simulink model "hexapod2"  (R2015a)
settings: Solver=ode23tb  StartTime=0.0  StopTime=10  FixedStep=0.0001  MaxStep=0.01  RelTol=1e-4  AbsTol=1e-5
values from neighbouring files (symbols this model uses):
  bH = 1    [runFirst.m]
  C = CM + CL/n^2    (= 0.0001377500155)    [runFirst.m]
  d1 = 0    [runFirst.m]    (also in runFirst2.m)
  d2 = -4.61    [runFirst.m]    (also in runFirst2.m = 0)
  J = JM + JL/n^2    (= 0.008455500031)    [runFirst.m]
  Ka = 12    [runFirst.m]
  Kb = 0.00867    [runFirst.m]
  Ke = 1    [runFirst.m]
  Km = 4.375    [runFirst.m]
  L = 0.0006    [runFirst.m]
  L1 = 3.64    [runFirst.m]    (also in runFirst2.m = 3.4)
  L2 = 5.72    [runFirst.m]    (also in runFirst2.m = 8.7)
  L3 = 12.46    [runFirst.m]    (also in runFirst2.m = 12.73)
  n = 254    [runFirst.m]
  R = 1.4    [runFirst.m]
undefined symbols (not defined in the file or in its folder): bLb, bLs, X, Y, Z
libraries: sm_lib x108, nesl_utility x43, simulink x24, Contact_Forces_Lib x7, roblocks x2
(part 1 of 5)
settings Model: Creator=340DANILOV  LastModifiedBy=340DANILOV
settings SolverCC: ZeroCrossAlgorithm=Adaptive
settings DataIOCC: LimitDataPoints=off  ReturnWorkspaceOutputs=on
settings DebuggingCC: IgnoredZcDiagnostic=none  SolverPrmCheckMsg=warning  UnconnectedInputMsg=none  UnconnectedOutputMsg=none
settings DiagnosticsConfigSet: SimMechanicsRigidlyBoundBlock=none

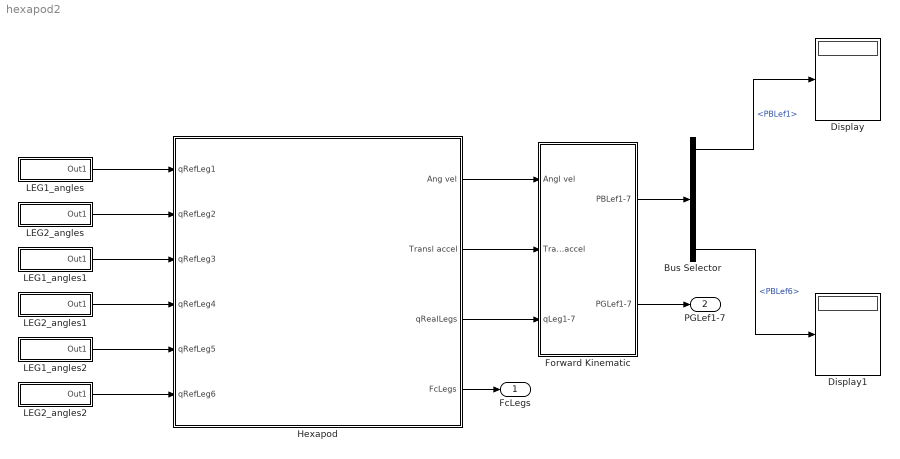
== system hexapod2 ==
  Bus Selector : BusSelector  OutputSignals=PBLef1,PBLef2,PBLef3,PBLef4,PBLef5,PBLef6
  Display : Display
  Display1 : Display
  Forward Kinematic : Subsystem
  Hexapod : Subsystem  mask(Hexapod model){}
      mask help:
      | This model describes hexapod robot with six insect legs. This model contain mechanics and servos.
      | You can change mass and size charasteristics of body and legs.
      | As a location is used a flat surface.
      |
      | Inputs:
      |  - qRefLeg<1...6> - reference angles for each leg.
      |             It is must be 1x3 massive with angles for each joint of leg.
      |
      | Outputs:
      |  - Ang vel - Angular velocities of CoM. Imitation of data from gyroscope.
      |  - Transl accel - CoM translation acceleration. Imitation of data from accelerometer.
      |  - FcLegs - Contact forces of end effectors each leg. It is 1x6 massive. Each element contains value for contact force each leg. Imitation of force sensors.
      |  - qRealLegs - Real angles of each link of hexapod legs. It is 3x6 massive. Imitation of data from servo encoder.
      mask Display:
      | image(imread('hexapod.png'))
      | 
      | 
      | port_label('output',1,'Ang vel')
      | port_label('output',2,'Transl accel')
      | port_label('output',3,'qRealLegs')
      | port_label('output',4,'FcLegs')
      | 
      | port_label('input',1,'qRefLeg1')
      | port_label('input',2,'qRefLeg2')
      | port_label('input',3,'qRefLeg3')
      | port_label('input',4,'qRefLeg4')
      | port_label('input',5,'qRefLeg5')
      | port_label('input',6,'qRefLeg6')
  LEG1_angles : Subsystem
  LEG1_angles1 : Subsystem
  LEG1_angles2 : Subsystem
  LEG2_angles : Subsystem
  LEG2_angles1 : Subsystem
  LEG2_angles2 : Subsystem
  FcLegs : Outport
  PGLef1-7 : Outport  Port=2
  wires:
  Hexapod/4(FcLegs) -> FcLegs/1
  Hexapod/1(Ang vel) -> Forward Kinematic/1(Angl vel)
  Hexapod/2(Transl accel) -> Forward Kinematic/2(Transl accel)
  Hexapod/3(qRealLegs) -> Forward Kinematic/3(qLeg1-7)
  Forward Kinematic/1(PBLef1-7) -> Bus Selector/1
  Forward Kinematic/2(PGLef1-7) -> PGLef1-7/1
  Bus Selector/1 -> Display/1  "<PBLef1>"
  Bus Selector/6 -> Display1/1  "<PBLef6>"
  LEG1_angles/1(Out1) -> Hexapod/1(qRefLeg1)
  LEG2_angles/1(Out1) -> Hexapod/2(qRefLeg2)
  LEG2_angles1/1(Out1) -> Hexapod/4(qRefLeg4)
  LEG2_angles2/1(Out1) -> Hexapod/6(qRefLeg6)
  LEG1_angles1/1(Out1) -> Hexapod/3(qRefLeg3)
  LEG1_angles2/1(Out1) -> Hexapod/5(qRefLeg5)

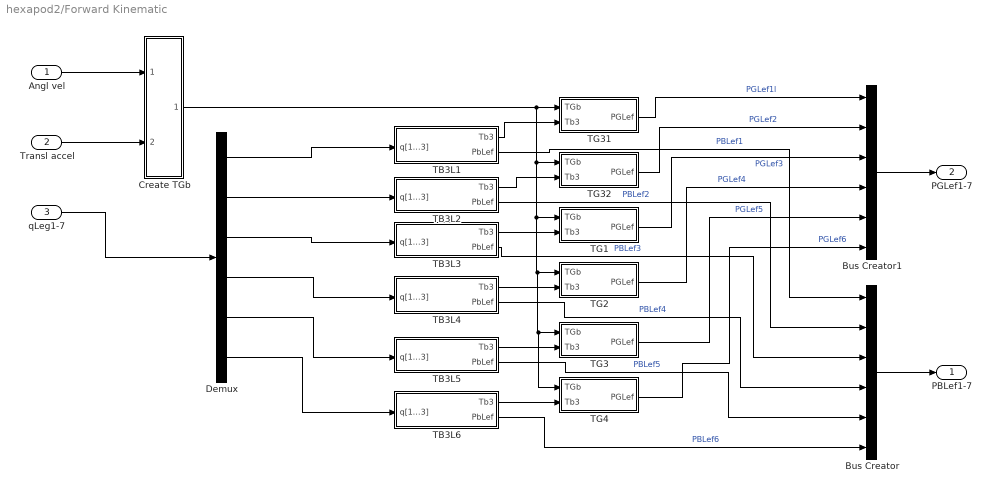
== system hexapod2/Forward Kinematic ==
  Angl vel : Inport
  Transl accel : Inport  Port=2
  qLeg1-7 : Inport  Port=3
  Bus Creator : BusCreator  Inputs=6
  Bus Creator1 : BusCreator  Inputs=6
  Create TGb : Subsystem
  Demux : Demux  Outputs=6
  TB3L1 : Subsystem
  TB3L2 : Subsystem
  TB3L3 : Subsystem
  TB3L4 : Subsystem
  TB3L5 : Subsystem
  TB3L6 : Subsystem
  TG1 : Subsystem
  TG2 : Subsystem
  TG3 : Subsystem
  TG31 : Subsystem
  TG32 : Subsystem
  TG4 : Subsystem
  PBLef1-7 : Outport
  PGLef1-7 : Outport  Port=2
  wires:
  Bus Creator/1 -> PBLef1-7/1
  TB3L6/1(Tb3) -> TG4/2(Tb3)
  TB3L5/2(PbLef) -> Bus Creator/5  "PBLef5"
  TB3L4/2(PbLef) -> Bus Creator/4  "PBLef4"
  TG3/1(PGLef) -> Bus Creator1/5  "PGLef5"
  TB3L6/2(PbLef) -> Bus Creator/6  "PBLef6"
  Demux/1 -> TB3L1/1(q[1...3])
  TB3L1/2(PbLef) -> Bus Creator/1  "PBLef1"
  Demux/6 -> TB3L6/1(q[1...3])
  TB3L1/1(Tb3) -> TG31/2(Tb3)
  Create TGb/1(Out1) -> TG4/1(TGb), TG3/1(TGb), TG2/1(TGb), TG1/1(TGb), TG32/1(TGb), TG31/1(TGb)
  Demux/4 -> TB3L4/1(q[1...3])
  Demux/3 -> TB3L3/1(q[1...3])
  TG31/1(PGLef) -> Bus Creator1/1  "PGLef1l"
  Demux/5 -> TB3L5/1(q[1...3])
  TB3L2/2(PbLef) -> Bus Creator/2  "PBLef2"
  TB3L2/1(Tb3) -> TG32/2(Tb3)
  TG32/1(PGLef) -> Bus Creator1/2  "PGLef2"
  TB3L4/1(Tb3) -> TG2/2(Tb3)
  TB3L3/1(Tb3) -> TG1/2(Tb3)
  TG1/1(PGLef) -> Bus Creator1/3  "PGLef3"
  Bus Creator1/1 -> PGLef1-7/1
  Angl vel/1 -> Create TGb/1(In1)
  Transl accel/1 -> Create TGb/2(In2)
  TB3L3/2(PbLef) -> Bus Creator/3  "PBLef3"
  qLeg1-7/1 -> Demux/1
  TB3L5/1(Tb3) -> TG3/2(Tb3)
  TG4/1(PGLef) -> Bus Creator1/6  "PGLef6"
  TG2/1(PGLef) -> Bus Creator1/4  "PGLef4"
  Demux/2 -> TB3L2/1(q[1...3])

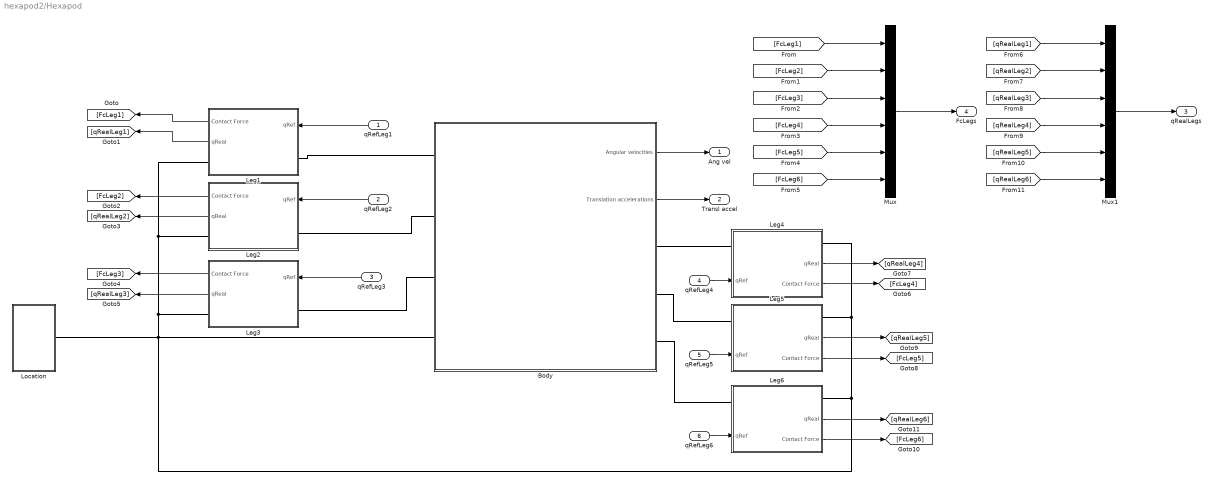
== system hexapod2/Hexapod ==
  qRefLeg1 : Inport
  qRefLeg2 : Inport  Port=2
  qRefLeg3 : Inport  Port=3
  qRefLeg4 : Inport  Port=4
  qRefLeg5 : Inport  Port=5
  qRefLeg6 : Inport  Port=6
  Body : Subsystem  mask(Hexapod Body){L=18.5, w1=10.5, w2=12.5, H=1, m=5, Z1Angle=45, Z2Angle=0, Z3Angle=-45, Z4Angle=-45, Z5Angle=0, Z6Angle=45}
      mask prompts: L "Length (cm)"; w1 "Small weigth (cm)"; w2 "Big weigth (cm)"; H "Heigth (cm)"; m "Mass (kg)"; Z1Angle "Leg1 Rotation"; Z2Angle "Leg2 Rotation"; Z3Angle "Leg3 Rotation"; Z4Angle "Leg4 Rotation"; Z5Angle "Leg5 Rotation"; Z6Angle "Leg6 Rotation"
      mask help: This block describes overall size, mass and reference frames of hexapod body.
      mask Display:
      | image(imread('body.png'))
      | text(5,10, 'Hexapod Body')
      | port_label('LConn',1,'Leg1')
      | port_label('LConn',2,'Leg2')
      | port_label('LConn',3,'Leg3')
      | port_label('LConn',4,'Global System')
      | port_label('RConn',1,'Leg4')
      | port_label('RConn',2,'Leg5')
      | port_label('RConn',3,'Leg6')
      | port_label('output',1,'Ang vel')
      | port_label('output',2,'Transl accel')
  Leg1 : Subsystem  mask(Insect leg){L1=L1, L2=L2, L3=L3, m1=0.1, m2=0.1, m3=0.1}
      mask prompts: L1 "Length 1 (cm)"; L2 "Lengh 2 (cm)"; L3 "Length 3 (cm)"; m1 "Mass 1 (kg)"; m2 "Mass 2 (kg)"; m3 "Mass 3(kg)"
      mask help: This block describes link length and their mass of the hexapod insect leg.
      mask Display:
      | image(imread('insect_leg.png'))
      | text(5,10, 'Insect leg')
      | port_label('LConn',1,'T0')
      | port_label('RConn',1,'Base')
      | port_label('input',1,'qRef')
      | port_label('output',1,'Fc')
      | port_label('output',2,'qReal')
  Leg2 : Subsystem  mask(Insect leg){L1=3.53, L2=5.7, L3=12.6, m1=0.1, m2=0.1, m3=0.1}
      mask prompts: L1 "Length 1 (cm)"; L2 "Lengh 2 (cm)"; L3 "Length 3 (cm)"; m1 "Mass 1 (kg)"; m2 "Mass 2 (kg)"; m3 "Mass 3(kg)"
      mask help: This block describes link length and their mass of the hexapod insect leg.
      mask Display:
      | image(imread('insect_leg.png'))
      | text(5,10, 'Insect leg')
      | port_label('LConn',1,'T0')
      | port_label('RConn',1,'Base')
      | port_label('input',1,'qRef')
      | port_label('output',1,'Fc')
      | port_label('output',2,'qReal')
  Leg3 : Subsystem  mask(Insect leg){L1=3.53, L2=5.7, L3=12.6, m1=0.1, m2=0.1, m3=0.1}
      mask prompts: L1 "Length 1 (cm)"; L2 "Lengh 2 (cm)"; L3 "Length 3 (cm)"; m1 "Mass 1 (kg)"; m2 "Mass 2 (kg)"; m3 "Mass 3(kg)"
      mask help: This block describes link length and their mass of the hexapod insect leg.
      mask Display:
      | image(imread('insect_leg.png'))
      | text(5,10, 'Insect leg')
      | port_label('LConn',1,'T0')
      | port_label('RConn',1,'Base')
      | port_label('input',1,'qRef')
      | port_label('output',1,'Fc')
      | port_label('output',2,'qReal')
  Leg4 : Subsystem  mask(Insect leg){L1=3.53, L2=5.7, L3=12.6, m1=0.1, m2=0.1, m3=0.1}
      mask prompts: L1 "Length 1 (cm)"; L2 "Lengh 2 (cm)"; L3 "Length 3 (cm)"; m1 "Mass 1 (kg)"; m2 "Mass 2 (kg)"; m3 "Mass 3(kg)"
      mask help: This block describes link length and their mass of the hexapod insect leg.
      mask Display:
      | image(imread('insect_leg.png'))
      | text(5,10, 'Insect leg')
      | port_label('LConn',1,'T0')
      | port_label('RConn',1,'Base')
      | port_label('input',1,'qRef')
      | port_label('output',1,'Fc')
      | port_label('output',2,'qReal')
  Leg5 : Subsystem  mask(Insect leg){L1=3.53, L2=5.7, L3=12.6, m1=0.1, m2=0.1, m3=0.1}
      mask prompts: L1 "Length 1 (cm)"; L2 "Lengh 2 (cm)"; L3 "Length 3 (cm)"; m1 "Mass 1 (kg)"; m2 "Mass 2 (kg)"; m3 "Mass 3(kg)"
      mask help: This block describes link length and their mass of the hexapod insect leg.
      mask Display:
      | image(imread('insect_leg.png'))
      | text(5,10, 'Insect leg')
      | port_label('LConn',1,'T0')
      | port_label('RConn',1,'Base')
      | port_label('input',1,'qRef')
      | port_label('output',1,'Fc')
      | port_label('output',2,'qReal')
  Leg6 : Subsystem  mask(Insect leg){L1=3.53, L2=5.7, L3=12.6, m1=0.1, m2=0.1, m3=0.1}
      mask prompts: L1 "Length 1 (cm)"; L2 "Lengh 2 (cm)"; L3 "Length 3 (cm)"; m1 "Mass 1 (kg)"; m2 "Mass 2 (kg)"; m3 "Mass 3(kg)"
      mask help: This block describes link length and their mass of the hexapod insect leg.
      mask Display:
      | image(imread('insect_leg.png'))
      | text(5,10, 'Insect leg')
      | port_label('LConn',1,'T0')
      | port_label('RConn',1,'Base')
      | port_label('input',1,'qRef')
      | port_label('output',1,'Fc')
      | port_label('output',2,'qReal')
  Location : Subsystem
  Mux : Mux  Inputs=6
  Mux1 : Mux  Inputs=6
  Ang vel : Outport
  Transl accel : Outport  Port=2
  qRealLegs : Outport  Port=3
  FcLegs : Outport  Port=4
  wires:
  qRefLeg1/1 -> Leg1/1(qRef)
  qRefLeg2/1 -> Leg2/1(qRef)
  qRefLeg3/1 -> Leg3/1(qRef)
  qRefLeg4/1 -> Leg4/1(qRef)
  Leg2/2(qReal) -> [qRealLeg2]
  Leg3/2(qReal) -> [qRealLeg3]
  Leg3/1(Contact Force) -> [FcLeg3]
  [FcLeg2] -> Mux/2
  [FcLeg4] -> Mux/4
  [FcLeg5] -> Mux/5
  [FcLeg1] -> Mux/1
  [FcLeg3] -> Mux/3
  [FcLeg6] -> Mux/6
  Mux/1 -> FcLegs/1
  Leg1/1(Contact Force) -> [FcLeg1]
  [qRealLeg4] -> Mux1/4
  [qRealLeg6] -> Mux1/6
  [qRealLeg2] -> Mux1/2
  [qRealLeg1] -> Mux1/1
  Mux1/1 -> qRealLegs/1
  [qRealLeg5] -> Mux1/5
  [qRealLeg3] -> Mux1/3
  Body/1(Angular velocities) -> Ang vel/1
  Body/2(Translation accelerations) -> Transl accel/1
  Leg1/2(qReal) -> [qRealLeg1]
  Leg2/1(Contact Force) -> [FcLeg2]
  qRefLeg5/1 -> Leg5/1(qRef)
  qRefLeg6/1 -> Leg6/1(qRef)
  Leg4/1(Contact Force) -> [FcLeg4]
  Leg4/2(qReal) -> [qRealLeg4]
  Leg5/2(qReal) -> [qRealLeg5]
  Leg5/1(Contact Force) -> [FcLeg5]
  Leg6/2(qReal) -> [qRealLeg6]
  Leg6/1(Contact Force) -> [FcLeg6]
  connections:
  Body/LConn1 -- Leg1/LConn1
  Body/LConn4 -- Leg6/RConn1 -- Leg5/RConn1 -- Leg4/RConn1 -- Location/RConn1 -- Leg3/RConn1 -- Leg2/RConn1 -- Leg1/RConn1
  Leg2/LConn1 -- Body/LConn2
  Leg3/LConn1 -- Body/LConn3
  Leg4/LConn1 -- Body/RConn1
  Leg5/LConn1 -- Body/RConn2
  Leg6/LConn1 -- Body/RConn3

== system hexapod2/LEG1_angles ==
  Clock : Clock
  Mux : Mux  Inputs=3
  Switch : Switch  Threshold=6
  leg1_theta2 : simulink/Sources/Repeating Sequence  rep_seq_t=[0 3 4 5 6]  rep_seq_y=[0 0 60*pi/180 60*pi/180 0]
  leg1_theta3 : simulink/Sources/Repeating Sequence  rep_seq_t=[0 3 4 5 6]  rep_seq_y=[0 0 60*pi/180 60*pi/180 0]
  theta1 : simulink/Sources/Repeating Sequence Interpolated  OutValues=[0 0 0 45*pi/180 45*pi/180].'  TimeValues=[0 3 4 5 6].'  LookUpMeth=Interpolation-Use End Values  tsamp=0.01  OutMin=[]  OutMax=[]  OutDataTypeStr=double  OutputDataTypeScalingMode=double  OutDataType=fixdt(0,8)  OutScaling=2^-10
  theta21 : simulink/Sources/Repeating Sequence Interpolated  OutValues=[45*pi/180 -45*pi/180 -45*pi/180 45*pi/180 45*pi/180].'  TimeValues=[0 3 4 5 6].'  LookUpMeth=Interpolation-Use End Values  tsamp=0.01  OutMin=[]  OutMax=[]  OutDataTypeStr=double  OutputDataTypeScalingMode=double  OutDataType=fixdt(0,8)  OutScaling=2^-10
  Out1 : Outport
  wires:
  theta1/1 -> Switch/3
  theta21/1 -> Switch/1
  Switch/1 -> Mux/1
  Clock/1 -> Switch/2
  Mux/1 -> Out1/1
  leg1_theta3/1 -> Mux/3
  leg1_theta2/1 -> Mux/2

== system hexapod2/LEG1_angles1 ==
  Clock : Clock
  Mux : Mux  Inputs=3
  Switch : Switch  Threshold=6
  leg1_theta2 : simulink/Sources/Repeating Sequence  rep_seq_t=[0 3 4 5 6]  rep_seq_y=[0 0 60*pi/180 60*pi/180 0]
  leg1_theta3 : simulink/Sources/Repeating Sequence  rep_seq_t=[0 3 4 5 6]  rep_seq_y=[0 0 60*pi/180 60*pi/180 0]
  theta1 : simulink/Sources/Repeating Sequence Interpolated  OutValues=[0 0 0 45*pi/180 45*pi/180].'  TimeValues=[0 3 4 5 6].'  LookUpMeth=Interpolation-Use End Values  tsamp=0.01  OutMin=[]  OutMax=[]  OutDataTypeStr=double  OutputDataTypeScalingMode=double  OutDataType=fixdt(0,8)  OutScaling=2^-10
  theta21 : simulink/Sources/Repeating Sequence Interpolated  OutValues=[45*pi/180 -45*pi/180 -45*pi/180 45*pi/180 45*pi/180].'  TimeValues=[0 3 4 5 6].'  LookUpMeth=Interpolation-Use End Values  tsamp=0.01  OutMin=[]  OutMax=[]  OutDataTypeStr=double  OutputDataTypeScalingMode=double  OutDataType=fixdt(0,8)  OutScaling=2^-10
  Out1 : Outport
  wires:
  leg1_theta2/1 -> Mux/2
  leg1_theta3/1 -> Mux/3
  Mux/1 -> Out1/1
  Clock/1 -> Switch/2
  Switch/1 -> Mux/1
  theta21/1 -> Switch/1
  theta1/1 -> Switch/3

== system hexapod2/LEG1_angles2 ==
  Clock : Clock
  Mux : Mux  Inputs=3
  Switch : Switch  Threshold=6
  leg1_theta2 : simulink/Sources/Repeating Sequence  rep_seq_t=[0 3 4 5 6]  rep_seq_y=[0 0 60*pi/180 60*pi/180 0]
  leg1_theta3 : simulink/Sources/Repeating Sequence  rep_seq_t=[0 3 4 5 6]  rep_seq_y=[0 0 60*pi/180 60*pi/180 0]
  theta1 : simulink/Sources/Repeating Sequence Interpolated  OutValues=[0 0 0 45*pi/180 45*pi/180].'  TimeValues=[0 3 4 5 6].'  LookUpMeth=Interpolation-Use End Values  tsamp=0.01  OutMin=[]  OutMax=[]  OutDataTypeStr=double  OutputDataTypeScalingMode=double  OutDataType=fixdt(0,8)  OutScaling=2^-10
  theta21 : simulink/Sources/Repeating Sequence Interpolated  OutValues=[45*pi/180 -45*pi/180 -45*pi/180 45*pi/180 45*pi/180].'  TimeValues=[0 3 4 5 6].'  LookUpMeth=Interpolation-Use End Values  tsamp=0.01  OutMin=[]  OutMax=[]  OutDataTypeStr=double  OutputDataTypeScalingMode=double  OutDataType=fixdt(0,8)  OutScaling=2^-10
  Out1 : Outport
  wires:
  theta1/1 -> Switch/3
  theta21/1 -> Switch/1
  Switch/1 -> Mux/1
  Clock/1 -> Switch/2
  Mux/1 -> Out1/1
  leg1_theta3/1 -> Mux/3
  leg1_theta2/1 -> Mux/2

== system hexapod2/LEG2_angles ==
  Clock : Clock
  Mux1 : Mux  Inputs=3
  Switch : Switch  Threshold=6
  leg2_theta2 : simulink/Sources/Repeating Sequence  rep_seq_t=[0 1 2 3 6]  rep_seq_y=[0 60*pi/180 60*pi/180 0 0]
  leg2_theta3 : simulink/Sources/Repeating Sequence  rep_seq_t=[0 1 2 3 6]  rep_seq_y=[0 60*pi/180 60*pi/180 0 0]
  theta1 : simulink/Sources/Repeating Sequence Interpolated  OutValues=[0 0 45*pi/180 45*pi/180 -45*pi/180].'  TimeValues=[0 1 2 3 6].'  LookUpMeth=Interpolation-Use End Values  tsamp=0.01  OutMin=[]  OutMax=[]  OutDataTypeStr=double  OutputDataTypeScalingMode=double  OutDataType=fixdt(0,8)  OutScaling=2^-10
  theta21 : simulink/Sources/Repeating Sequence Interpolated  OutValues=[-45*pi/180 -45*pi/180 45*pi/180 45*pi/180 -45*pi/180].'  TimeValues=[0 1 2 3 6].'  LookUpMeth=Interpolation-Use End Values  tsamp=0.01  OutMin=[]  OutMax=[]  OutDataTypeStr=double  OutputDataTypeScalingMode=double  OutDataType=fixdt(0,8)  OutScaling=2^-10
  Out1 : Outport
  wires:
  Switch/1 -> Mux1/1
  theta1/1 -> Switch/3
  theta21/1 -> Switch/1
  Clock/1 -> Switch/2
  leg2_theta2/1 -> Mux1/2
  leg2_theta3/1 -> Mux1/3
  Mux1/1 -> Out1/1

== system hexapod2/LEG2_angles1 ==
  Clock : Clock
  Mux1 : Mux  Inputs=3
  Switch : Switch  Threshold=6
  leg2_theta2 : simulink/Sources/Repeating Sequence  rep_seq_t=[0 1 2 3 6]  rep_seq_y=[0 60*pi/180 60*pi/180 0 0]
  leg2_theta3 : simulink/Sources/Repeating Sequence  rep_seq_t=[0 1 2 3 6]  rep_seq_y=[0 60*pi/180 60*pi/180 0 0]
  theta1 : simulink/Sources/Repeating Sequence Interpolated  OutValues=[0 0 45*pi/180 45*pi/180 -45*pi/180].'  TimeValues=[0 1 2 3 6].'  LookUpMeth=Interpolation-Use End Values  tsamp=0.01  OutMin=[]  OutMax=[]  OutDataTypeStr=double  OutputDataTypeScalingMode=double  OutDataType=fixdt(0,8)  OutScaling=2^-10
  theta21 : simulink/Sources/Repeating Sequence Interpolated  OutValues=[-45*pi/180 -45*pi/180 45*pi/180 45*pi/180 -45*pi/180].'  TimeValues=[0 1 2 3 6].'  LookUpMeth=Interpolation-Use End Values  tsamp=0.01  OutMin=[]  OutMax=[]  OutDataTypeStr=double  OutputDataTypeScalingMode=double  OutDataType=fixdt(0,8)  OutScaling=2^-10
  Out1 : Outport
  wires:
  Mux1/1 -> Out1/1
  leg2_theta3/1 -> Mux1/3
  leg2_theta2/1 -> Mux1/2
  Clock/1 -> Switch/2
  theta21/1 -> Switch/1
  theta1/1 -> Switch/3
  Switch/1 -> Mux1/1

== system hexapod2/LEG2_angles2 ==
  Clock : Clock
  Mux1 : Mux  Inputs=3
  Switch : Switch  Threshold=6
  leg2_theta2 : simulink/Sources/Repeating Sequence  rep_seq_t=[0 1 2 3 6]  rep_seq_y=[0 60*pi/180 60*pi/180 0 0]
  leg2_theta3 : simulink/Sources/Repeating Sequence  rep_seq_t=[0 1 2 3 6]  rep_seq_y=[0 60*pi/180 60*pi/180 0 0]
  theta1 : simulink/Sources/Repeating Sequence Interpolated  OutValues=[0 0 45*pi/180 45*pi/180 -45*pi/180].'  TimeValues=[0 1 2 3 6].'  LookUpMeth=Interpolation-Use End Values  tsamp=0.01  OutMin=[]  OutMax=[]  OutDataTypeStr=double  OutputDataTypeScalingMode=double  OutDataType=fixdt(0,8)  OutScaling=2^-10
  theta21 : simulink/Sources/Repeating Sequence Interpolated  OutValues=[-45*pi/180 -45*pi/180 45*pi/180 45*pi/180 -45*pi/180].'  TimeValues=[0 1 2 3 6].'  LookUpMeth=Interpolation-Use End Values  tsamp=0.01  OutMin=[]  OutMax=[]  OutDataTypeStr=double  OutputDataTypeScalingMode=double  OutDataType=fixdt(0,8)  OutScaling=2^-10
  Out1 : Outport
  wires:
  Switch/1 -> Mux1/1
  theta1/1 -> Switch/3
  theta21/1 -> Switch/1
  Clock/1 -> Switch/2
  leg2_theta2/1 -> Mux1/2
  leg2_theta3/1 -> Mux1/3
  Mux1/1 -> Out1/1

== system hexapod2/Forward Kinematic/Create TGb ==
  note: TBG
  In1 : Inport
  In2 : Inport  Port=2
  Demux : Demux  Outputs=3
  Demux1 : Demux  Outputs=3
  Integrator : Integrator
  Integrator1 : Integrator
  Integrator2 : Integrator
  Product : Product  Multiplication=Matrix(*)
  Switch1 : Subsystem
  Switch2 : Subsystem
  Transfer Fcn : TransferFcn  Denominator=[1 0 0]
  Transfer Fcn1 : TransferFcn  Denominator=[1 0 0]
  Transfer Fcn2 : TransferFcn  Denominator=[1 0 0]
  rpy2T : roblocks/Transform Conversion/rpy2T
      link override MATLAB Fcn: MATLABFcn=rpy2tr(u(1),u(2),u(3))
  xyz2T : roblocks/Transform Conversion/xyz2T
  Out1 : Outport
  wires:
  Integrator1/1 -> rpy2T/2
  Integrator2/1 -> rpy2T/3
  Integrator/1 -> rpy2T/1
  Switch2/1(Out1) -> Demux1/1
  In2/1 -> Switch2/1(In1)
  In1/1 -> Switch1/1(In1)
  Switch1/1(Out1) -> Demux/1
  Transfer Fcn/1 -> xyz2T/1
  Transfer Fcn1/1 -> xyz2T/2
  Transfer Fcn2/1 -> xyz2T/3
  Demux1/3 -> Transfer Fcn2/1
  Demux1/1 -> Transfer Fcn/1
  Demux/3 -> Integrator2/1
  Demux1/2 -> Transfer Fcn1/1
  Product/1 -> Out1/1
  xyz2T/1 -> Product/2
  rpy2T/1 -> Product/1
  Demux/2 -> Integrator1/1
  Demux/1 -> Integrator/1

== system hexapod2/Forward Kinematic/TB3L1 ==
  note: Tb3
  note: PBL1ef
  q[1...3] : Inport
  Constant : Constant  Value=[L3; 0; 0; 1]  VectorParams1D=off
  Demux2 : Demux
  Mux : Mux  Inputs=3
  Product1 : Product  Multiplication=Matrix(*)
  Product2 : Product  Multiplication=Matrix(*)
  T30 : Subsystem
  Tbleg1 : Constant  Value=[cos(45*pi/180) -sin(45*pi/180) 0 bH/2; sin(45*pi/180) cos(45*pi/180) 0 bLs/2; 0 0 1 0; 0 0 0 1]  VectorParams1D=off
  Terminator : Terminator
  Tb3 : Outport
  PbLef : Outport  Port=2
  wires:
  Constant/1 -> Product1/2
  q[1...3]/1 -> T30/1(In1)
  T30/1(Out1) -> Product2/2
  Tbleg1/1 -> Product2/1
  Demux2/3 -> Mux/3
  Product1/1 -> Demux2/1
  Demux2/4 -> Terminator/1
  Demux2/1 -> Mux/1
  Mux/1 -> PbLef/1
  Demux2/2 -> Mux/2
  Product2/1 -> Tb3/1, Product1/1

== system hexapod2/Forward Kinematic/TB3L2 ==
  note: PBL1ef
  note: Tb3
  q[1...3] : Inport
  Constant : Constant  Value=[L3; 0; 0; 1]  VectorParams1D=off
  Demux2 : Demux
  Mux : Mux  Inputs=3
  Product1 : Product  Multiplication=Matrix(*)
  Product2 : Product  Multiplication=Matrix(*)
  T30 : Subsystem
  Tbleg1 : Constant  Value=[0 -1 0 0; 1 0 0 bLb/2; 0 0 1 0; 0 0 0 1]  VectorParams1D=off
  Terminator : Terminator
  Tb3 : Outport
  PbLef : Outport  Port=2
  wires:
  Product2/1 -> Product1/1, Tb3/1
  Demux2/2 -> Mux/2
  Mux/1 -> PbLef/1
  Demux2/1 -> Mux/1
  Demux2/4 -> Terminator/1
  Product1/1 -> Demux2/1
  Demux2/3 -> Mux/3
  Tbleg1/1 -> Product2/1
  T30/1(Out1) -> Product2/2
  q[1...3]/1 -> T30/1(In1)
  Constant/1 -> Product1/2

== system hexapod2/Forward Kinematic/TB3L3 ==
  note: Tb3
  note: PBL1ef
  q[1...3] : Inport
  Constant : Constant  Value=[L3; 0; 0; 1]  VectorParams1D=off
  Demux2 : Demux
  Mux : Mux  Inputs=3
  Product1 : Product  Multiplication=Matrix(*)
  Product2 : Product  Multiplication=Matrix(*)
  T30 : Subsystem
  Tbleg3 : Constant  Value=[cos(135*pi/180) -sin(135*pi/180) 0 -bH/2; sin(135*pi/180) cos(135*pi/180) 0 bLs/2; 0 0 1 0; 0 0 0 1]  VectorParams1D=off
  Terminator : Terminator
  Tb3 : Outport
  PbLef : Outport  Port=2
  wires:
  Constant/1 -> Product1/2
  q[1...3]/1 -> T30/1(In1)
  T30/1(Out1) -> Product2/2
  Tbleg3/1 -> Product2/1
  Demux2/3 -> Mux/3
  Product1/1 -> Demux2/1
  Demux2/4 -> Terminator/1
  Demux2/1 -> Mux/1
  Mux/1 -> PbLef/1
  Demux2/2 -> Mux/2
  Product2/1 -> Tb3/1, Product1/1

== system hexapod2/Forward Kinematic/TB3L4 ==
  note: PBL1ef
  note: Tb3
  q[1...3] : Inport
  Constant : Constant  Value=[L3; 0; 0; 1]  VectorParams1D=off
  Demux2 : Demux
  Mux : Mux  Inputs=3
  Product1 : Product  Multiplication=Matrix(*)
  Product2 : Product  Multiplication=Matrix(*)
  T30 : Subsystem
  Tbleg1 : Constant  Value=[cos(-45*pi/180) -sin(-45*pi/180) 0 bH/2; sin(-45*pi/180) cos(-45*pi/180) 0 -bLs/2; 0 0 1 0; 0 0 0 1]  VectorParams1D=off
  Terminator : Terminator
  Tb3 : Outport
  PbLef : Outport  Port=2
  wires:
  Product2/1 -> Product1/1, Tb3/1
  Demux2/2 -> Mux/2
  Mux/1 -> PbLef/1
  Demux2/1 -> Mux/1
  Demux2/4 -> Terminator/1
  Product1/1 -> Demux2/1
  Demux2/3 -> Mux/3
  Tbleg1/1 -> Product2/1
  T30/1(Out1) -> Product2/2
  q[1...3]/1 -> T30/1(In1)
  Constant/1 -> Product1/2

== system hexapod2/Forward Kinematic/TB3L5 ==
  note: Tb3
  note: PBL1ef
  q[1...3] : Inport
  Constant : Constant  Value=[L3; 0; 0; 1]  VectorParams1D=off
  Demux2 : Demux
  Mux : Mux  Inputs=3
  Product1 : Product  Multiplication=Matrix(*)
  Product2 : Product  Multiplication=Matrix(*)
  T30 : Subsystem
  Tbleg1 : Constant  Value=[0 1 0 0; -1 0 0 -bLb/2; 0 0 1 0; 0 0 0 1]  VectorParams1D=off
  Terminator : Terminator
  Tb3 : Outport
  PbLef : Outport  Port=2
  wires:
  Constant/1 -> Product1/2
  q[1...3]/1 -> T30/1(In1)
  T30/1(Out1) -> Product2/2
  Tbleg1/1 -> Product2/1
  Demux2/3 -> Mux/3
  Product1/1 -> Demux2/1
  Demux2/4 -> Terminator/1
  Demux2/1 -> Mux/1
  Mux/1 -> PbLef/1
  Demux2/2 -> Mux/2
  Product2/1 -> Tb3/1, Product1/1

== system hexapod2/Forward Kinematic/TB3L6 ==
  note: Tb3
  note: PBL1ef
  q[1...3] : Inport
  Constant : Constant  Value=[L3; 0; 0; 1]  VectorParams1D=off
  Demux2 : Demux
  Mux : Mux  Inputs=3
  Product1 : Product  Multiplication=Matrix(*)
  Product2 : Product  Multiplication=Matrix(*)
  T30 : Subsystem
  Tbleg1 : Constant  Value=[cos(-135*pi/180) -sin(-135*pi/180) 0 -bH/2; sin(-135*pi/180) cos(-135*pi/180) 0 -bLs/2; 0 0 1 0; 0 0 0 1]  VectorParams1D=off
  Terminator : Terminator
  Tb3 : Outport
  PbLef : Outport  Port=2
  wires:
  Constant/1 -> Product1/2
  q[1...3]/1 -> T30/1(In1)
  T30/1(Out1) -> Product2/2
  Tbleg1/1 -> Product2/1
  Demux2/3 -> Mux/3
  Product1/1 -> Demux2/1
  Demux2/4 -> Terminator/1
  Demux2/1 -> Mux/1
  Mux/1 -> PbLef/1
  Demux2/2 -> Mux/2
  Product2/1 -> Tb3/1, Product1/1

== system hexapod2/Forward Kinematic/TG1 ==
  note: PGL1ef
  TGb : Inport
  Tb3 : Inport  Port=2
  Constant1 : Constant  Value=[0; L3; 0; 1]  VectorParams1D=off
  Demux1 : Demux
  Mux1 : Mux  Inputs=3
  Product3 : Product  Multiplication=Matrix(*)
  Product4 : Product  Multiplication=Matrix(*)
  Terminator1 : Terminator
  PGLef : Outport
  wires:
  Tb3/1 -> Product3/2
  Demux1/2 -> Mux1/2
  Demux1/4 -> Terminator1/1
  Demux1/3 -> Mux1/3
  Mux1/1 -> PGLef/1
  Product4/1 -> Demux1/1
  Demux1/1 -> Mux1/1
  Constant1/1 -> Product4/2
  TGb/1 -> Product3/1
  Product3/1 -> Product4/1

== system hexapod2/Forward Kinematic/TG2 ==
  note: PGL1ef
  TGb : Inport
  Tb3 : Inport  Port=2
  Constant1 : Constant  Value=[0; L3; 0; 1]  VectorParams1D=off
  Demux1 : Demux
  Mux1 : Mux  Inputs=3
  Product3 : Product  Multiplication=Matrix(*)
  Product4 : Product  Multiplication=Matrix(*)
  Terminator1 : Terminator
  PGLef : Outport
  wires:
  Product3/1 -> Product4/1
  TGb/1 -> Product3/1
  Constant1/1 -> Product4/2
  Demux1/1 -> Mux1/1
  Product4/1 -> Demux1/1
  Mux1/1 -> PGLef/1
  Demux1/3 -> Mux1/3
  Demux1/4 -> Terminator1/1
  Demux1/2 -> Mux1/2
  Tb3/1 -> Product3/2

== system hexapod2/Forward Kinematic/TG3 ==
  note: PGL1ef
  TGb : Inport
  Tb3 : Inport  Port=2
  Constant1 : Constant  Value=[0; L3; 0; 1]  VectorParams1D=off
  Demux1 : Demux
  Mux1 : Mux  Inputs=3
  Product3 : Product  Multiplication=Matrix(*)
  Product4 : Product  Multiplication=Matrix(*)
  Terminator1 : Terminator
  PGLef : Outport
  wires:
  Tb3/1 -> Product3/2
  Demux1/2 -> Mux1/2
  Demux1/4 -> Terminator1/1
  Demux1/3 -> Mux1/3
  Mux1/1 -> PGLef/1
  Product4/1 -> Demux1/1
  Demux1/1 -> Mux1/1
  Constant1/1 -> Product4/2
  TGb/1 -> Product3/1
  Product3/1 -> Product4/1

== system hexapod2/Forward Kinematic/TG31 ==
  note: PGL1ef
  TGb : Inport
  Tb3 : Inport  Port=2
  Constant1 : Constant  Value=[0; L3; 0; 1]  VectorParams1D=off
  Demux1 : Demux
  Mux1 : Mux  Inputs=3
  Product3 : Product  Multiplication=Matrix(*)
  Product4 : Product  Multiplication=Matrix(*)
  Terminator1 : Terminator
  PGLef : Outport
  wires:
  Tb3/1 -> Product3/2
  Demux1/2 -> Mux1/2
  Demux1/4 -> Terminator1/1
  Demux1/3 -> Mux1/3
  Mux1/1 -> PGLef/1
  Product4/1 -> Demux1/1
  Demux1/1 -> Mux1/1
  Constant1/1 -> Product4/2
  TGb/1 -> Product3/1
  Product3/1 -> Product4/1

== system hexapod2/Forward Kinematic/TG32 ==
  note: PGL1ef
  TGb : Inport
  Tb3 : Inport  Port=2
  Constant1 : Constant  Value=[0; L3; 0; 1]  VectorParams1D=off
  Demux1 : Demux
  Mux1 : Mux  Inputs=3
  Product3 : Product  Multiplication=Matrix(*)
  Product4 : Product  Multiplication=Matrix(*)
  Terminator1 : Terminator
  PGLef : Outport
  wires:
  Product3/1 -> Product4/1
  TGb/1 -> Product3/1
  Constant1/1 -> Product4/2
  Demux1/1 -> Mux1/1
  Product4/1 -> Demux1/1
  Mux1/1 -> PGLef/1
  Demux1/3 -> Mux1/3
  Demux1/4 -> Terminator1/1
  Demux1/2 -> Mux1/2
  Tb3/1 -> Product3/2

== system hexapod2/Forward Kinematic/TG4 ==
  note: PGL1ef
  TGb : Inport
  Tb3 : Inport  Port=2
  Constant1 : Constant  Value=[0; L3; 0; 1]  VectorParams1D=off
  Demux1 : Demux
  Mux1 : Mux  Inputs=3
  Product3 : Product  Multiplication=Matrix(*)
  Product4 : Product  Multiplication=Matrix(*)
  Terminator1 : Terminator
  PGLef : Outport
  wires:
  Tb3/1 -> Product3/2
  Demux1/2 -> Mux1/2
  Demux1/4 -> Terminator1/1
  Demux1/3 -> Mux1/3
  Mux1/1 -> PGLef/1
  Product4/1 -> Demux1/1
  Demux1/1 -> Mux1/1
  Constant1/1 -> Product4/2
  TGb/1 -> Product3/1
  Product3/1 -> Product4/1

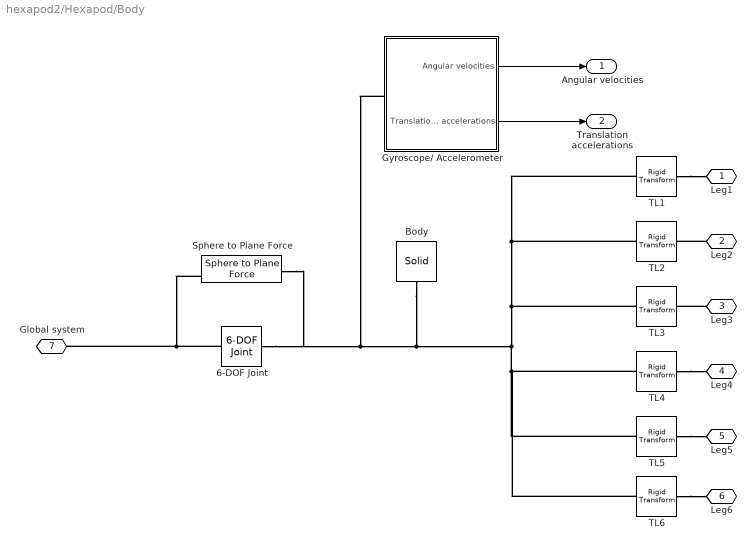
== system hexapod2/Hexapod/Body ==
  6-DOF Joint : sm_lib/Joints/6-DOF Joint  SenseConstraintForce=off  SenseConstraintForceX=off  SenseConstraintForceY=off  SenseConstraintForceZ=off  SenseConstraintTorque=off  SenseConstraintTorqueX=off  SenseConstraintTorqueY=off  SenseConstraintTorqueZ=off  SenseTotalForce=off  SenseTotalForceX=off  SenseTotalForceY=off  SenseTotalForceZ=off  SenseTotalTorque=off  SenseTotalTorqueX=off  SenseTotalTorqueY=off  SenseTotalTorqueZ=off  CompositeWrenchDir=FollowerOnBase  CompositeWrenchFrame=BaseFrame  PxEquilibriumPosition=0  PxEquilibriumPositionUnits=m  PxSpringStiffness=0  PxSpringStiffnessUnits=N/m  PxDampingCoefficient=0  PxDampingCoefficientUnits=N/(m/s)  PxTorqueActuationMode=NoTorque  PxMotionActuationMode=ComputedMotion  PxSensePosition=off  PxSenseVelocity=off  PxSenseAcceleration=off  PxSenseTorqueForce=off  PxPositionTargetSpecify=off  PxPositionTargetPriority=High  PxPositionTargetValue=0.5  PxPositionTargetValueUnits=m  PxVelocityTargetSpecify=off  PxVelocityTargetPriority=High  PxVelocityTargetValue=0.5  PxVelocityTargetValueUnits=m/s  PyEquilibriumPosition=0  PyEquilibriumPositionUnits=m  PySpringStiffness=0  PySpringStiffnessUnits=N/m  PyDampingCoefficient=0  PyDampingCoefficientUnits=N/(m/s)  PyTorqueActuationMode=NoTorque  PyMotionActuationMode=ComputedMotion  PySensePosition=off  PySenseVelocity=off  PySenseAcceleration=off  PySenseTorqueForce=off  PyPositionTargetSpecify=off  PyPositionTargetPriority=High  PyPositionTargetValue=0  PyPositionTargetValueUnits=m  PyVelocityTargetSpecify=off  PyVelocityTargetPriority=High  PyVelocityTargetValue=0  PyVelocityTargetValueUnits=m/s  PzEquilibriumPosition=0  PzEquilibriumPositionUnits=m  PzSpringStiffness=0  PzSpringStiffnessUnits=N/m  PzDampingCoefficient=0  PzDampingCoefficientUnits=N/(m/s)  PzTorqueActuationMode=NoTorque  PzMotionActuationMode=ComputedMotion  PzSensePosition=off  PzSenseVelocity=off  PzSenseAcceleration=off  PzSenseTorqueForce=off  PzPositionTargetSpecify=on  PzPositionTargetPriority=High  PzPositionTargetValue=0.2  PzPositionTargetValueUnits=m  PzVelocityTargetSpecify=off  PzVelocityTargetPriority=High  PzVelocityTargetValue=0  PzVelocityTargetValueUnits=m/s  SphDefPosRotationMethod=None  SphDefPosRotationAngleUnits=deg  SphDefPosRotationStandardAxis=+Z  SphDefPosRotationAngle=0.0  SphDefPosRotationArbitraryAxis=[0 0 1]  SphDefPosFollAlignAxisA=+X  SphDefPosBaseAlignAxisA=+Y  SphDefPosFollAlignAxisB=+Y  SphDefPosBaseAlignAxisB=+Z  SphDefPosRotationMatrix=[1 0 0; 0 1 0; 0 0 1]  SphEqPosRotationMethod=None  SphEqPosRotationAngleUnits=deg  SphEqPosRotationStandardAxis=+Z  SphEqPosRotationAngle=0.0  SphEqPosRotationArbitraryAxis=[0 0 1]  SphEqPosFollAlignAxisA=+X  SphEqPosBaseAlignAxisA=+Y  SphEqPosFollAlignAxisB=+Y  SphEqPosBaseAlignAxisB=+Z  SphEqPosRotationMatrix=[1 0 0; 0 1 0; 0 0 1]  SphSpringStiffness=0  SphSpringStiffnessUnits=N*m/deg  SphDampingCoefficient=0  SphDampingCoefficientUnits=N*m/(deg/s)  SphActuateTorqueX=off  SphActuateTorqueY=off  SphActuateTorqueZ=off  SphActuateTorque=off  SphTorqueActuationMode=NoTorque  SphMotionActuationMode=ComputedMotion  SphActuationFrame=BaseFrame  SphSensePosition=off  SphSenseVelocityX=off  SphSenseVelocityY=off  SphSenseVelocityZ=off  SphSenseVelocity=off  SphSenseAccelerationX=off  SphSenseAccelerationY=off  SphSenseAccelerationZ=off  SphSenseAcceleration=off  SphSenseTorqueX=off  SphSenseTorqueY=off  SphSenseTorqueZ=off  SphSenseTorqueForce=off  SphSensingFrame=BaseFrame  SphPositionTargetRotationMethod=None  SphPositionTargetRotationAngleUnits=deg  SphPositionTargetRotationStandardAxis=+Z  SphPositionTargetRotationAngle=0.0  SphPositionTargetRotationArbitraryAxis=[0 0 1]  SphPositionTargetFollAlignAxisA=+X  SphPositionTargetBaseAlignAxisA=+Y  SphPositionTargetFollAlignAxisB=+Y  SphPositionTargetBaseAlignAxisB=+Z  SphPositionTargetRotationMatrix=[1 0 0; 0 1 0; 0 0 1]  SphPositionTargetSpecify=off  SphPositionTargetPriority=High  SphVelocityTargetValue=[0 0 0]  SphVelocityTargetValueUnits=deg/s  SphVelocityTargetSpecify=off  SphVelocityTargetPriority=High  SphVelocityTargetInFollowerFrame=on  BlockFunction=simmechanics.library.joints.sixdof_joint
  Body : sm_lib/Body Elements/Solid  InertiaType=CalculateFromGeometry  Mass=m  MassUnits=kg  CenterOfMass=[0 0 0]  CenterOfMassUnits=m  MomentsOfInertia=[1 1 1]  MomentsOfInertiaUnits=kg*m^2  ProductsOfInertia=[0 0 0]  ProductsOfInertiaUnits=kg*m^2  DensityBased=off  Density=5000  DensityUnits=kg/(m^3)  GraphicType=FromGeometry  MarkerShape=Sphere  MarkerSize=10  MarkerSizeUnits=m  GraphicVisPropType=SimpleVisualProperties  GraphicDiffuseColor=[0.0 0.4 0.0]  GraphicSpecularColor=[0.5 0.5 0.5 1.0]  GraphicAmbientColor=[0.15 0.15 0.15 1.0]  GraphicEmissiveColor=[0.0 0.0 0.0 1.0]  GraphicShininess=75  GraphicOpacity=1.0  GeometryShape=GeneralExtrusion  RectangleSize=[1 1]  RectangleSizeUnits=m  BrickDimensions=[18.5 12.5 1]  BrickDimensionUnits=cm  CylinderRadius=1  CylinderRadiusUnits=m  CylinderLength=1  CylinderLengthUnits=m  SphereRadius=1  SphereRadiusUnits=m  EllipsoidRadii=[1 1 1]  EllipsoidRadiiUnits=m  ExtrusionCrossSection=[L/2 w1/2; 0 w2/2; -L/2 w1/2; -L/2 -w1/2; 0 -w2/2; L/2 -w1/2]  ExtrusionCrossSectionUnits=cm  ExtrusionLength=H  ExtrusionLengthUnits=cm  PolygonNumSides=3  PolygonOuterRadius=1  PolygonOuterRadiusUnits=m  ExtGeomFileType=STL  ExtGeomFileUnits=m  RevolutionCrossSection=[1 1; 1 -1; 2 -1; 2 1]  RevolutionCrossSectionUnits=m  RevolutionExtent=Full  RevolutionAngle=180  RevolutionAngleUnits=deg  BlockFunction=simmechanics.library.body_elements.solid
  Gyroscope/ Accelerometer : Subsystem
  Sphere to Plane Force : Contact_Forces_Lib/3D/Sphere to Plane Force  sphere_rad=0.005  plane_lenx=2  plane_leny=2  plane_depth=0.01/2  force_law=Linear  k_contact=1e7  b_contact=1e4  pen_full_damp_F=1e-4  pen_exponent=1  custom_param_1=1  custom_param_2=1  friction_law=Stick-Slip Continuous  mu_kinetic=0.5  mu_static=0.7  v_thr=0.001
  TL1 : sm_lib/Frames and Transforms/Rigid Transform  TranslationMethod=Cartesian  TranslationLengthUnit=cm  TranslationStandardAxis=+Z  TranslationStandardOffset=0  TranslationCartesianOffset=[L/2 w1/2 0]  TranslationROffset=0  TranslationROffsetUnits=m  TranslationZOffset=0  TranslationZOffsetUnits=m  TranslationThetaOffset=0  TranslationThetaOffsetUnits=deg  RotationMethod=StandardAxis  RotationAngleUnits=deg  RotationStandardAxis=+Z  RotationAngle=90-Z1Angle  RotationArbitraryAxis=[0 0 1]  FollAlignAxisA=+X  BaseAlignAxisA=+Y  FollAlignAxisB=+Y  BaseAlignAxisB=+Z  RotationMatrix=[1 0 0; 0 1 0; 0 0 1]  BlockFunction=simmechanics.library.frames_transforms.rigid_transform
  TL2 : sm_lib/Frames and Transforms/Rigid Transform  TranslationMethod=Cartesian  TranslationLengthUnit=cm  TranslationStandardAxis=+Z  TranslationStandardOffset=0  TranslationCartesianOffset=[0 w2/2 0]  TranslationROffset=0  TranslationROffsetUnits=m  TranslationZOffset=0  TranslationZOffsetUnits=m  TranslationThetaOffset=0  TranslationThetaOffsetUnits=deg  RotationMethod=StandardAxis  RotationAngleUnits=deg  RotationStandardAxis=+Z  RotationAngle=90-Z2Angle  RotationArbitraryAxis=[0 0 1]  FollAlignAxisA=+X  BaseAlignAxisA=+Y  FollAlignAxisB=+Y  BaseAlignAxisB=+Z  RotationMatrix=[1 0 0; 0 1 0; 0 0 1]  BlockFunction=simmechanics.library.frames_transforms.rigid_transform
  TL3 : sm_lib/Frames and Transforms/Rigid Transform  TranslationMethod=Cartesian  TranslationLengthUnit=cm  TranslationStandardAxis=+Z  TranslationStandardOffset=0  TranslationCartesianOffset=[-L/2 w1/2 0]  TranslationROffset=0  TranslationROffsetUnits=m  TranslationZOffset=0  TranslationZOffsetUnits=m  TranslationThetaOffset=0  TranslationThetaOffsetUnits=deg  RotationMethod=StandardAxis  RotationAngleUnits=deg  RotationStandardAxis=+Z  RotationAngle=90-Z3Angle  RotationArbitraryAxis=[0 0 1]  FollAlignAxisA=+X  BaseAlignAxisA=+Y  FollAlignAxisB=+Y  BaseAlignAxisB=+Z  RotationMatrix=[1 0 0; 0 1 0; 0 0 1]  BlockFunction=simmechanics.library.frames_transforms.rigid_transform
  TL4 : sm_lib/Frames and Transforms/Rigid Transform  TranslationMethod=Cartesian  TranslationLengthUnit=cm  TranslationStandardAxis=+Z  TranslationStandardOffset=0  TranslationCartesianOffset=[L/2 -w1/2 0]  TranslationROffset=0  TranslationROffsetUnits=m  TranslationZOffset=0  TranslationZOffsetUnits=m  TranslationThetaOffset=0  TranslationThetaOffsetUnits=deg  RotationMethod=StandardAxis  RotationAngleUnits=deg  RotationStandardAxis=+Z  RotationAngle=-90-Z4Angle  RotationArbitraryAxis=[0 0 1]  FollAlignAxisA=+X  BaseAlignAxisA=+Y  FollAlignAxisB=+Y  BaseAlignAxisB=+Z  RotationMatrix=[1 0 0; 0 1 0; 0 0 1]  BlockFunction=simmechanics.library.frames_transforms.rigid_transform
  TL5 : sm_lib/Frames and Transforms/Rigid Transform  TranslationMethod=Cartesian  TranslationLengthUnit=cm  TranslationStandardAxis=+Z  TranslationStandardOffset=0  TranslationCartesianOffset=[0 -w2/2 0]  TranslationROffset=0  TranslationROffsetUnits=m  TranslationZOffset=0  TranslationZOffsetUnits=m  TranslationThetaOffset=0  TranslationThetaOffsetUnits=deg  RotationMethod=StandardAxis  RotationAngleUnits=deg  RotationStandardAxis=+Z  RotationAngle=-90-Z5Angle  RotationArbitraryAxis=[0 0 1]  FollAlignAxisA=+X  BaseAlignAxisA=+Y  FollAlignAxisB=+Y  BaseAlignAxisB=+Z  RotationMatrix=[1 0 0; 0 1 0; 0 0 1]  BlockFunction=simmechanics.library.frames_transforms.rigid_transform
  TL6 : sm_lib/Frames and Transforms/Rigid Transform  TranslationMethod=Cartesian  TranslationLengthUnit=cm  TranslationStandardAxis=+Z  TranslationStandardOffset=0  TranslationCartesianOffset=[-L/2 -w1/2 0]  TranslationROffset=0  TranslationROffsetUnits=m  TranslationZOffset=0  TranslationZOffsetUnits=m  TranslationThetaOffset=0  TranslationThetaOffsetUnits=deg  RotationMethod=StandardAxis  RotationAngleUnits=deg  RotationStandardAxis=+Z  RotationAngle=-90-Z6Angle  RotationArbitraryAxis=[0 0 1]  FollAlignAxisA=+X  BaseAlignAxisA=+Y  FollAlignAxisB=+Y  BaseAlignAxisB=+Z  RotationMatrix=[1 0 0; 0 1 0; 0 0 1]  BlockFunction=simmechanics.library.frames_transforms.rigid_transform
  Leg1 : PMIOPort  Port=1  Side=Left
  Leg2 : PMIOPort  Port=2  Side=Left
  Leg3 : PMIOPort  Port=3  Side=Left
  Leg4 : PMIOPort  Port=4  Side=Right
  Leg5 : PMIOPort  Port=5  Side=Right
  Leg6 : PMIOPort  Port=6  Side=Right
  Global system : PMIOPort  Port=7  Side=Left
  Angular velocities : Outport
  Translation accelerations : Outport  Port=2
  wires:
  Gyroscope/ Accelerometer/1(Angular velocities) -> Angular velocities/1
  Gyroscope/ Accelerometer/2(Translation accelerations) -> Translation accelerations/1
  connections:
  TL1/RConn1 -- Leg1/RConn1
  Leg2/RConn1 -- TL2/RConn1
  Leg3/RConn1 -- TL3/RConn1
  TL4/RConn1 -- Leg4/RConn1
  TL5/RConn1 -- Leg5/RConn1
  TL6/RConn1 -- Leg6/RConn1
  TL1/LConn1 -- Gyroscope/ Accelerometer/LConn1 -- Sphere to Plane Force/LConn1 -- 6-DOF Joint/RConn1 -- Body/RConn1 -- TL6/LConn1 -- TL5/LConn1 -- TL4/LConn1 -- TL3/LConn1 -- TL2/LConn1
  6-DOF Joint/LConn1 -- Sphere to Plane Force/RConn1 -- Global system/RConn1

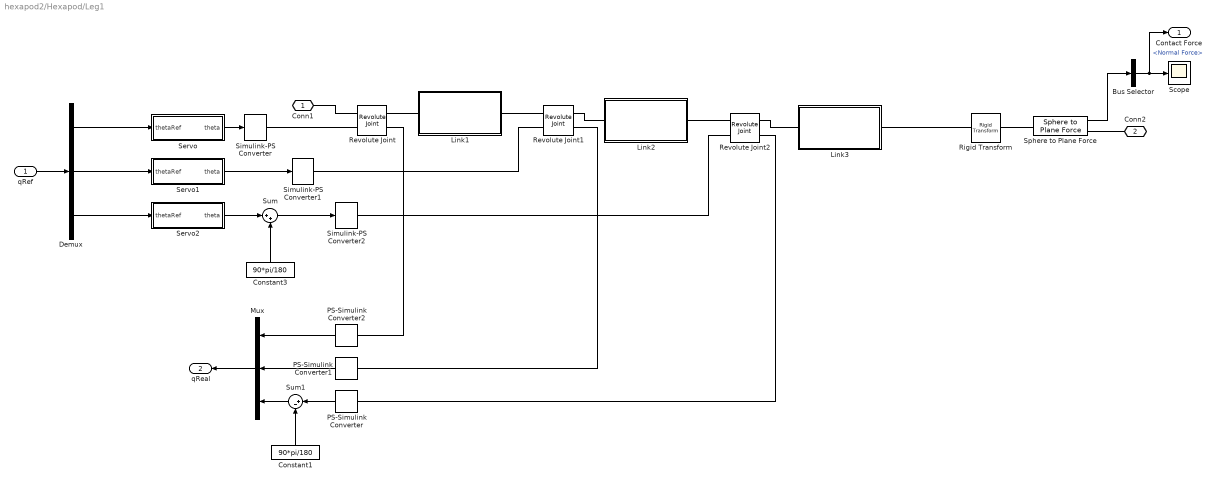
== system hexapod2/Hexapod/Leg1 ==
  qRef : Inport
  Bus Selector : BusSelector  OutputSignals=Normal Force
  Constant1 : Constant  Value=90*pi/180
  Constant3 : Constant  Value=90*pi/180
  Demux : Demux  Outputs=3
  Link1 : Subsystem  mask{L=L1, W=1, H=1, m=m1, rgb=[0.1 0.1 0.90], Xangle=90, d1=-2.3}
      mask prompts: L "Length (cm)"; W "Width (cm)"; H "Thickness (cm)"; m "Mass (kg)"; rgb "Color [R G B]"; Xangle "+X Rotation (deg)"
      mask Display:
      | text(5,10, 'Link')
      | image(imread('sm_smpl_body.png'))
      | port_label('LConn',1,'L')
      | port_label('RConn',1,'R')
  Link2 : Subsystem  mask{L=L2, W=1, H=1, m=m2, rgb=[0.1 0.9 0.1], Xangle=180}
      mask prompts: L "Length (cm)"; W "Width (cm)"; H "Thickness (cm)"; m "Mass (kg)"; rgb "Color [R G B]"; Xangle "+X Rotation (deg)"
      mask Display:
      | text(5,10, 'Link')
      | image(imread('sm_smpl_body.png'))
      | port_label('LConn',1,'L')
      | port_label('RConn',1,'R')
  Link3 : Subsystem  mask{L=L3, W=1, H=1, m=m3, rgb=[0.9 0.1 0.10], Xangle=0}
      mask prompts: L "Length (cm)"; W "Width (cm)"; H "Thickness (cm)"; m "Mass (kg)"; rgb "Color [R G B]"; Xangle "+X Rotation (deg)"
      mask Display:
      | text(5,10, 'Link')
      | image(imread('sm_smpl_body.png'))
      | port_label('LConn',1,'L')
      | port_label('RConn',1,'R')
  Mux : Mux  Inputs=3
  PS-Simulink Converter : nesl_utility/PS-Simulink Converter  PhysicalDomain=network_engine_domain  SubClassName=ps_output  LeftPortType=input  RightPortType=output  PseudoPeriodic=off  Frequencies=[]  Unit=1  AffineConversion=off
  PS-Simulink Converter1 : nesl_utility/PS-Simulink Converter  PhysicalDomain=network_engine_domain  SubClassName=ps_output  LeftPortType=input  RightPortType=output  PseudoPeriodic=off  Frequencies=[]  Unit=1  AffineConversion=off
  PS-Simulink Converter2 : nesl_utility/PS-Simulink Converter  PhysicalDomain=network_engine_domain  SubClassName=ps_output  LeftPortType=input  RightPortType=output  PseudoPeriodic=off  Frequencies=[]  Unit=1  AffineConversion=off
  Revolute Joint : sm_lib/Joints/Revolute Joint  SenseConstraintForce=off  SenseConstraintForceX=off  SenseConstraintForceY=off  SenseConstraintForceZ=off  SenseConstraintTorque=off  SenseConstraintTorqueX=off  SenseConstraintTorqueY=off  SenseConstraintTorqueZ=off  SenseTotalForce=off  SenseTotalForceX=off  SenseTotalForceY=off  SenseTotalForceZ=off  SenseTotalTorque=off  SenseTotalTorqueX=off  SenseTotalTorqueY=off  SenseTotalTorqueZ=off  CompositeWrenchDir=FollowerOnBase  CompositeWrenchFrame=BaseFrame  EquilibriumPosition=0  EquilibriumPositionUnits=deg  SpringStiffness=0  SpringStiffnessUnits=N*m/deg  DampingCoefficient=0  DampingCoefficientUnits=N*m/(deg/s)  TorqueActuationMode=ComputedTorque  MotionActuationMode=InputMotion  SensePosition=on  SenseVelocity=off  SenseAcceleration=off  SenseTorqueForce=off  PositionTargetSpecify=off  PositionTargetPriority=High  PositionTargetValue=0  PositionTargetValueUnits=deg  VelocityTargetSpecify=off  VelocityTargetPriority=High  VelocityTargetValue=0  VelocityTargetValueUnits=deg/s  BlockFunction=simmechanics.library.joints.revolute_joint
  Revolute Joint1 : sm_lib/Joints/Revolute Joint  SenseConstraintForce=off  SenseConstraintForceX=off  SenseConstraintForceY=off  SenseConstraintForceZ=off  SenseConstraintTorque=off  SenseConstraintTorqueX=off  SenseConstraintTorqueY=off  SenseConstraintTorqueZ=off  SenseTotalForce=off  SenseTotalForceX=off  SenseTotalForceY=off  SenseTotalForceZ=off  SenseTotalTorque=off  SenseTotalTorqueX=off  SenseTotalTorqueY=off  SenseTotalTorqueZ=off  CompositeWrenchDir=FollowerOnBase  CompositeWrenchFrame=BaseFrame  EquilibriumPosition=0  EquilibriumPositionUnits=deg  SpringStiffness=0  SpringStiffnessUnits=N*m/deg  DampingCoefficient=0  DampingCoefficientUnits=N*m/(deg/s)  TorqueActuationMode=ComputedTorque  MotionActuationMode=InputMotion  SensePosition=on  SenseVelocity=off  SenseAcceleration=off  SenseTorqueForce=off  PositionTargetSpecify=off  PositionTargetPriority=High  PositionTargetValue=0  PositionTargetValueUnits=deg  VelocityTargetSpecify=off  VelocityTargetPriority=High  VelocityTargetValue=0  VelocityTargetValueUnits=deg/s  BlockFunction=simmechanics.library.joints.revolute_joint
  Revolute Joint2 : sm_lib/Joints/Revolute Joint  SenseConstraintForce=off  SenseConstraintForceX=off  SenseConstraintForceY=off  SenseConstraintForceZ=off  SenseConstraintTorque=off  SenseConstraintTorqueX=off  SenseConstraintTorqueY=off  SenseConstraintTorqueZ=off  SenseTotalForce=off  SenseTotalForceX=off  SenseTotalForceY=off  SenseTotalForceZ=off  SenseTotalTorque=off  SenseTotalTorqueX=off  SenseTotalTorqueY=off  SenseTotalTorqueZ=off  CompositeWrenchDir=FollowerOnBase  CompositeWrenchFrame=BaseFrame  EquilibriumPosition=0  EquilibriumPositionUnits=deg  SpringStiffness=0  SpringStiffnessUnits=N*m/deg  DampingCoefficient=0  DampingCoefficientUnits=N*m/(deg/s)  TorqueActuationMode=ComputedTorque  MotionActuationMode=InputMotion  SensePosition=on  SenseVelocity=off  SenseAcceleration=off  SenseTorqueForce=off  PositionTargetSpecify=off  PositionTargetPriority=High  PositionTargetValue=0  PositionTargetValueUnits=deg  VelocityTargetSpecify=off  VelocityTargetPriority=High  VelocityTargetValue=0  VelocityTargetValueUnits=deg/s  BlockFunction=simmechanics.library.joints.revolute_joint
  Rigid Transform : sm_lib/Frames and Transforms/Rigid Transform  TranslationMethod=StandardAxis  TranslationLengthUnit=m  TranslationStandardAxis=-X  TranslationStandardOffset=0.01  TranslationCartesianOffset=[0 0 0]  TranslationROffset=0  TranslationROffsetUnits=m  TranslationZOffset=0  TranslationZOffsetUnits=m  TranslationThetaOffset=0  TranslationThetaOffsetUnits=deg  RotationMethod=None  RotationAngleUnits=deg  RotationStandardAxis=+Z  RotationAngle=0.0  RotationArbitraryAxis=[0 0 1]  FollAlignAxisA=+X  BaseAlignAxisA=+Y  FollAlignAxisB=+Y  BaseAlignAxisB=+Z  RotationMatrix=[1 0 0; 0 1 0; 0 0 1]  BlockFunction=simmechanics.library.frames_transforms.rigid_transform
  Scope : Scope
      settings: YMin=0  YMax=14000  SaveName=ScopeData7
  Servo : Subsystem
  Servo1 : Subsystem
  Servo2 : Subsystem
  Simulink-PS Converter : nesl_utility/Simulink-PS Converter  PhysicalDomain=network_engine_domain  SubClassName=ps_input  LeftPortType=input  RightPortType=output  PseudoPeriodic=off  Frequencies=[]  NoiseDistribution=none  NoiseParameters=[]  Unit=1  AffineConversion=off  InputFiltering=on  SimscapeFilterOrder=2  InputFilterTimeConstant=0.001  UdotUserProvided=1
  Simulink-PS Converter1 : nesl_utility/Simulink-PS Converter  PhysicalDomain=network_engine_domain  SubClassName=ps_input  LeftPortType=input  RightPortType=output  PseudoPeriodic=off  Frequencies=[]  NoiseDistribution=none  NoiseParameters=[]  Unit=1  AffineConversion=off  InputFiltering=on  SimscapeFilterOrder=2  InputFilterTimeConstant=0.001  UdotUserProvided=1
  Simulink-PS Converter2 : nesl_utility/Simulink-PS Converter  PhysicalDomain=network_engine_domain  SubClassName=ps_input  LeftPortType=input  RightPortType=output  PseudoPeriodic=off  Frequencies=[]  NoiseDistribution=none  NoiseParameters=[]  Unit=1  AffineConversion=off  InputFiltering=on  SimscapeFilterOrder=2  InputFilterTimeConstant=0.001  UdotUserProvided=1
  Sphere to Plane Force : Contact_Forces_Lib/3D/Sphere to Plane Force  sphere_rad=0.01  plane_lenx=2  plane_leny=2  plane_depth=0.01/2  force_law=Linear  k_contact=1e5  b_contact=1e4  pen_full_damp_F=1e-4  pen_exponent=1  custom_param_1=1  custom_param_2=1  friction_law=Stick-Slip Continuous  mu_kinetic=2  mu_static=2  v_thr=0.001
  Sum : Sum  Inputs=|++
  Sum1 : Sum  Inputs=|+-
  Conn1 : PMIOPort  Port=1  Side=Left
  Conn2 : PMIOPort  Port=2  Side=Right
  Contact Force : Outport
  qReal : Outport  Port=2
  wires:
  Demux/2 -> Servo1/1(thetaRef)
  Demux/3 -> Servo2/1(thetaRef)
  Sum/1 -> Simulink-PS Converter2/1
  Constant3/1 -> Sum/2
  Demux/1 -> Servo/1(thetaRef)
  qRef/1 -> Demux/1
  Servo/1(theta) -> Simulink-PS Converter/1
  Servo1/1(theta) -> Simulink-PS Converter1/1
  Servo2/1(theta) -> Sum/1
  Sphere to Plane Force/1 -> Bus Selector/1
  Bus Selector/1 -> Contact Force/1, Scope/1  "<Normal Force>"
  Mux/1 -> qReal/1
  PS-Simulink Converter2/1 -> Mux/1
  PS-Simulink Converter1/1 -> Mux/2
  PS-Simulink Converter/1 -> Sum1/1
  Sum1/1 -> Mux/3
  Constant1/1 -> Sum1/2
  connections:
  Link1/LConn1 -- Revolute Joint/RConn1
  Revolute Joint/LConn1 -- Conn1/RConn1
  Revolute Joint/LConn2 -- Simulink-PS Converter/RConn1
  Revolute Joint1/LConn1 -- Link1/RConn1
  Revolute Joint1/RConn1 -- Link2/LConn1
  Revolute Joint2/LConn1 -- Link2/RConn1
  Revolute Joint2/RConn1 -- Link3/LConn1
  Simulink-PS Converter1/RConn1 -- Revolute Joint1/LConn2
  Revolute Joint2/LConn2 -- Simulink-PS Converter2/RConn1
  Rigid Transform/LConn1 -- Link3/RConn1
  Sphere to Plane Force/LConn1 -- Rigid Transform/RConn1
  Conn2/RConn1 -- Sphere to Plane Force/RConn1
  PS-Simulink Converter/LConn1 -- Revolute Joint2/RConn2
  PS-Simulink Converter1/LConn1 -- Revolute Joint1/RConn2
  PS-Simulink Converter2/LConn1 -- Revolute Joint/RConn2
